simulink model "untitled"  (R2021a)
settings: Solver=VariableStepAuto  StartTime=0.0  StopTime=60  RelTol=1e-3
libraries: commrandsrc3 x4, simulink_extras x4
settings Model: Creator=PS  LastModifiedBy=PS

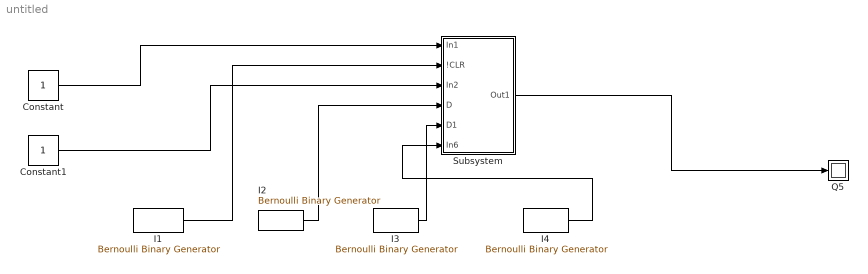
== system untitled ==
  Constant : Constant  OutDataTypeStr=boolean
  Constant1 : Constant  OutDataTypeStr=boolean
  I{1..4} (4 alike) : commrandsrc3/Bernoulli Binary Generator  ProbabilityOfZero=0.8  SeedSource=Auto  Seed=0  SampleTime=1  SamplesPerFrame=1  OutputDataType=boolean  SimulateUsing=Interpreted execution
  Q5 : Display
  Subsystem : Subsystem
  wires:
  Constant/1 -> Subsystem/1(In1)
  Constant1/1 -> Subsystem/3(In2)
  I1/1 -> Subsystem/2(!CLR)
  I2/1 -> Subsystem/4(D)
  I3/1 -> Subsystem/5(D1)
  I4/1 -> Subsystem/6(In6)
  Subsystem/1(Out1) -> Q5/1

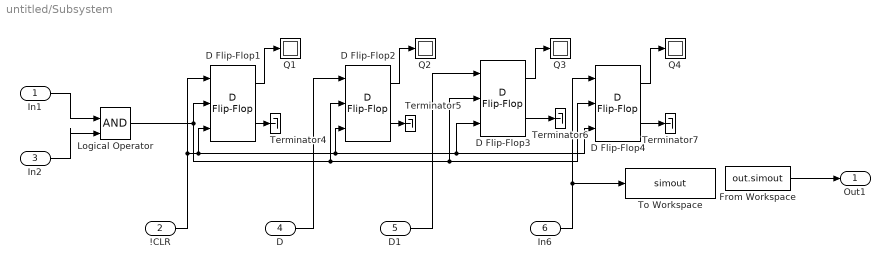
== system untitled/Subsystem ==
  In1 : Inport
  !CLR : Inport  Port=2
  In2 : Inport  Port=3
  D : Inport  Port=4
  D1 : Inport  Port=5
  In6 : Inport  Port=6
  D Flip-Flop{1..4} (4 alike) : simulink_extras/Flip Flops/D Flip-Flop
  From Workspace : FromWorkspace  VariableName=out.simout
  Logical Operator : Logic  IconShape=distinctive  AllPortsSameDT=off  OutDataTypeStr=boolean
  Q{1..4} (4 alike) : Display
  Terminator{4..7} (4 alike) : Terminator
  To Workspace : ToWorkspace  VariableName=simout  SaveFormat=Timeseries  SampleTime=-1
  Out1 : Outport
  wires:
  D1/1 -> D Flip-Flop3/1
  !CLR/1 -> D Flip-Flop1/3, D Flip-Flop4/3, D Flip-Flop3/3, D Flip-Flop2/3, D Flip-Flop1/1
  D Flip-Flop3/1 -> Q3/1
  Logical Operator/1 -> D Flip-Flop4/2, D Flip-Flop3/2, D Flip-Flop2/2, D Flip-Flop1/2
  D Flip-Flop3/2 -> Terminator6/1
  D Flip-Flop4/2 -> Terminator7/1
  In6/1 -> To Workspace/1, D Flip-Flop4/1
  D Flip-Flop2/1 -> Q2/1
  D Flip-Flop2/2 -> Terminator5/1
  D Flip-Flop1/2 -> Terminator4/1
  D Flip-Flop4/1 -> Q4/1
  D Flip-Flop1/1 -> Q1/1
  D/1 -> D Flip-Flop2/1
  In1/1 -> Logical Operator/1
  From Workspace/1 -> Out1/1
  In2/1 -> Logical Operator/2
